simulink model "Model_Automatique_BO_PI_enZ"  (R2020a)
settings: Solver=VariableStepAuto  StartTime=0.0  StopTime=tfinal  RelTol=1e-6
undefined symbols (not defined in the file or in its folder): tau3, tau4, Te
settings Model: Creator=mdescham  LastModifiedBy=mdescham

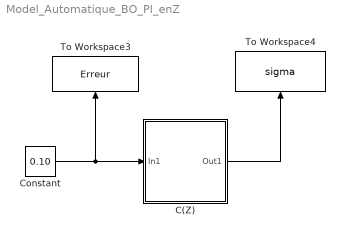
== system Model_Automatique_BO_PI_enZ ==
  C(Z) : Subsystem
  Constant : Constant  Value=0.10
  To Workspace3 : ToWorkspace  VariableName=Erreur  SaveFormat=Timeseries  SampleTime=-1
  To Workspace4 : ToWorkspace  VariableName=sigma  SaveFormat=Timeseries  SampleTime=-1
  wires:
  C(Z)/1(Out1) -> To Workspace4/1
  Constant/1 -> C(Z)/1(In1), To Workspace3/1

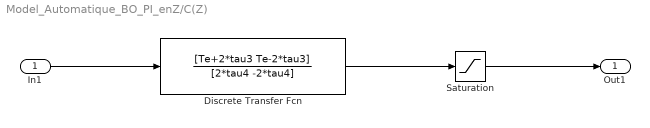
== system Model_Automatique_BO_PI_enZ/C(Z) ==
  In1 : Inport
  Discrete Transfer Fcn : DiscreteTransferFcn  Numerator=[Te+2*tau3 Te-2*tau3]  Denominator=[2*tau4 -2*tau4]  SampleTime=Te
  Saturation : Saturate  UpperLimit=0.45  LowerLimit=-0.45
  Out1 : Outport
  wires:
  In1/1 -> Discrete Transfer Fcn/1
  Discrete Transfer Fcn/1 -> Saturation/1
  Saturation/1 -> Out1/1
